simulink model "svpwm_sfunction"  (R2022a)
settings: Solver=ode23tb  StartTime=0.0  StopTime=0.05  FixedStep=10e-6  MaxStep=0.00001  RelTol=1e-3  EnableMultiTasking=on
InitFcn:
  | Vdc=700;
libraries: simulink_extras x1, simulink x1
settings Model: Creator=Administrator  LastModifiedBy=25313
settings SolverCC: AlgebraicLoopSolver=TrustRegion
settings DataIOCC: LimitDataPoints=on  SaveFormat=Array  SignalLoggingSaveFormat=ModelDataLogs  ReturnWorkspaceOutputs=off
settings OptimizationCC: ExpressionDepthLimit=2147483647  InitFltsAndDblsToZero=on  LifeSpan=inf
settings DebuggingCC: SaveWithParameterizedLinksMsg=none  UnderspecifiedInitializationDetection=Classic  MergeDetectMultiDrivingBlocksExec=none  SignalResolutionControl=TryResolveAllWithWarning  SolverPrmCheckMsg=warning  MultiTaskDSMMsg=warning  MultiTaskCondExecSysMsg=none  FcnCallInpInsideContextMsg=warning  UnconnectedInputMsg=warning  UnconnectedOutputMsg=warning  UnconnectedLineMsg=warning  StateNameClashWarn=warning  SFUnexpectedBacktrackingDiag=warning  SFNoUnconditionalDefaultTransitionDiag=warning  SFExecutionAtInitializationDiag=none  SFMachineParentedDataDiag=warning  ArithmeticOperatorsInVariantConditions=warning
settings HardwareCC: ProdBitPerPointer=32  ProdBitPerSizeT=32  ProdBitPerPtrDiffT=32  ProdLargestAtomicFloat=None  ProdIntDivRoundTo=Undefined  ProdEndianess=Unspecified  ProdWordSize=32  ProdHWDeviceType=32-bit Generic
settings ModelReferenceCC: PropagateSignalLabelsOutOfModel=off
settings SFSimCC: SimUseLocalCustomCode=off  CustomCodeUndefinedFunction=UseInterfaceOnly
settings RTWCC: RTWUseLocalCustomCode=off
settings CodeAppCC: StateflowObjectComments=on
settings GRTTargetCC: TargetFcnLib=ansi_tfl_tmw.mat  TargetLangStandard=C89/C90 (ANSI)  CombineOutputUpdateFcns=off  GRTInterface=on
settings ConfigComp: CovMetricSettings=dw  CovSaveCumulativeToWorkspaceVar=on  CovSaveSingleToWorkspaceVar=on  CovExternalEMLEnable=off

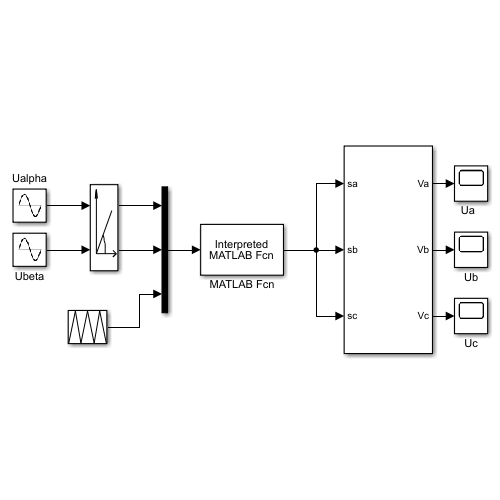
[thumbnail: Simulink's stored preview of the top-level diagram]
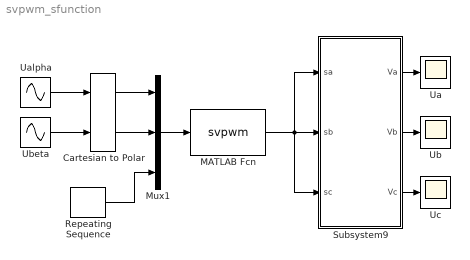
== system svpwm_sfunction ==
  Cartesian to Polar : simulink_extras/Transformations/Cartesian to Polar
  MATLAB Fcn : MATLABFcn  MATLABFcn=svpwm
  Mux1 : Mux  Inputs=3
  Repeating Sequence : simulink/Sources/Repeating Sequence  rep_seq_t=[0 0.0002 0.0004]  rep_seq_y=[0 0.0002 0]
  Subsystem9 : Subsystem
  "Ua  " : Scope
  Ualpha : Sin  Amplitude=200  Frequency=100*pi  Phase=pi/2  SampleTime=0
  Ub : Scope
  Ubeta : Sin  Amplitude=200  Frequency=100*pi  SampleTime=0
  Uc : Scope
  wires:
  Subsystem9/1(Va) -> "Ua  "/1
  Subsystem9/2(Vb) -> Ub/1
  Subsystem9/3(Vc) -> Uc/1
  Cartesian to Polar/1 -> Mux1/1
  Cartesian to Polar/2 -> Mux1/2
  Repeating Sequence/1 -> Mux1/3
  Mux1/1 -> MATLAB Fcn/1
  MATLAB Fcn/1 -> Subsystem9/3(sc), Subsystem9/1(sa), Subsystem9/2(sb)
  Ualpha/1 -> Cartesian to Polar/1
  Ubeta/1 -> Cartesian to Polar/2

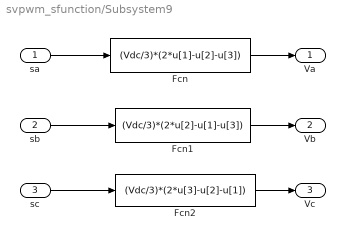
== system svpwm_sfunction/Subsystem9 ==
  sa : Inport
  sb : Inport  Port=2
  sc : Inport  Port=3
  Fcn : Fcn  Expr=(Vdc/3)*(2*u[1]-u[2]-u[3])
  Fcn1 : Fcn  Expr=(Vdc/3)*(2*u[2]-u[1]-u[3])
  Fcn2 : Fcn  Expr=(Vdc/3)*(2*u[3]-u[2]-u[1])
  Va : Outport
  Vb : Outport  Port=2
  Vc : Outport  Port=3
  wires:
  Fcn/1 -> Va/1
  Fcn1/1 -> Vb/1
  Fcn2/1 -> Vc/1
  sa/1 -> Fcn/1
  sb/1 -> Fcn1/1
  sc/1 -> Fcn2/1
